simulink model "Example_MultiPID"  (R2017b)
settings: Solver=FixedStepAuto  StartTime=0.0  StopTime=inf  FixedStep=0.01  RelTol=1e-3  EnableMultiTasking=on
libraries: OBD2_SocketCan_Library x1
settings Model: SimulationMode=external  Creator=Murml  LastModifiedBy=Murml
settings SolverCC: PositivePriorityOrder=on
settings OptimizationCC: PassReuseOutputArgsThreshold=0  MaxStackSize=64
settings DebuggingCC: ParameterTunabilityLossMsg=error
settings HardwareCC: ProdBitPerPointer=32  ProdBitPerSizeT=32  ProdBitPerPtrDiffT=32  ProdLargestAtomicInteger=Long  ProdLargestAtomicFloat=Double  ProdWordSize=32  ProdHWDeviceType=ARM Compatible->ARM Cortex  UseEmbeddedCoderFeatures=off
settings SFSimCC: MATLABDynamicMemAlloc=off
settings RTWCC: SystemTargetFile=ert.tlc  HardwareBoard=Raspberry Pi  TemplateMakefile=ert_default_tmf  Toolchain=GNU GCC Raspberry Pi
settings CodeAppCC: ForceParamTrailComments=on  OperatorAnnotations=on
settings ERTTargetCC: ERTCustomFileBanners=off  SupportContinuousTime=on  SupportNonInlinedSFcns=on  RemoveResetFunc=off  SupportVariableSizeSignals=on  ModelStepFunctionPrototypeControlCompliant=off

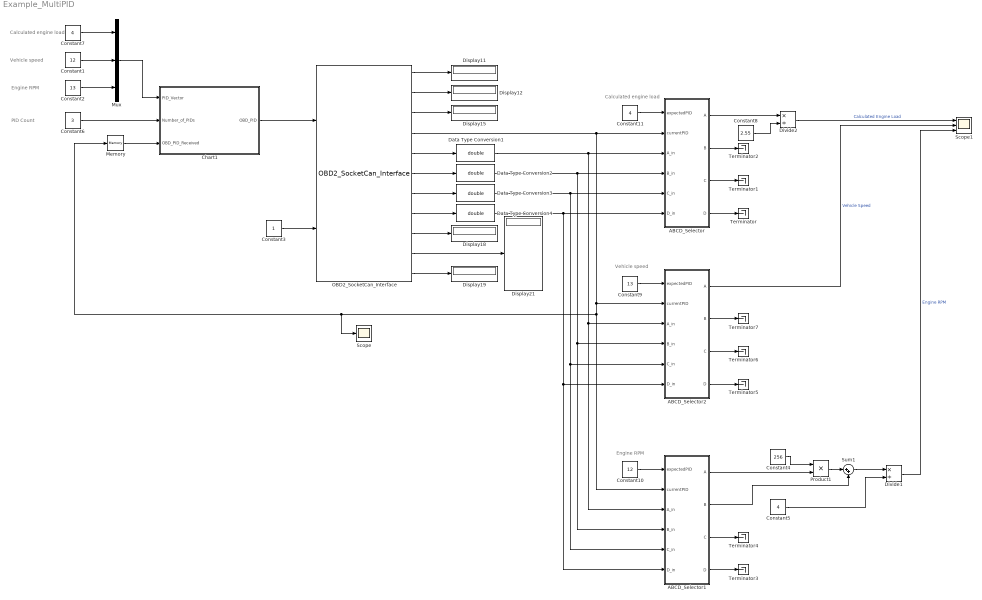
== system Example_MultiPID ==
  note: Calculated engine load
  note: Vehicle speed
  note: Engine RPM
  note: PID Count
  note: Calculated engine load
  note: Engine RPM
  note: Vehicle speed
  ABCD_Selector : MATLAB Function  TreatAsAtomicUnit=on
  ABCD_Selector1 : MATLAB Function  TreatAsAtomicUnit=on
  ABCD_Selector2 : MATLAB Function  TreatAsAtomicUnit=on
  Chart1 : Stateflow chart  TreatAsAtomicUnit=on
  Constant1 : Constant  Value=12  OutDataTypeStr=uint8  SampleTime=-1
  Constant10 : Constant  Value=12  OutDataTypeStr=uint8  SampleTime=-1
  Constant11 : Constant  Value=4  OutDataTypeStr=uint8  SampleTime=-1
  Constant2 : Constant  Value=13  OutDataTypeStr=uint8  SampleTime=-1
  Constant3 : Constant  OutDataTypeStr=uint8  SampleTime=-1
  Constant4 : Constant  Value=256  SampleTime=-1
  Constant5 : Constant  Value=4  SampleTime=-1
  Constant6 : Constant  Value=3  OutDataTypeStr=uint8  SampleTime=-1
  Constant7 : Constant  Value=4  OutDataTypeStr=uint8  SampleTime=-1
  Constant8 : Constant  Value=2.55  SampleTime=-1
  Constant9 : Constant  Value=13  OutDataTypeStr=uint8  SampleTime=-1
  Data Type Conversion{1..4} (4 alike) : DataTypeConversion  OutDataTypeStr=double
  Display{11..12,15,18..19,21} (6 alike) : Display
      Display11 settings: Format=hex (Stored Integer)
  Divide1 : Product  Inputs=*/
  Divide2 : Product  Inputs=*/
  Memory : Memory
  Mux : Mux  Inputs=3
  OBD2_SocketCan_Interface : OBD2_SocketCan_Library/OBD2_SocketCan_Interface  sampleTime=0.1
      settings: SourceProductName=OBD2 SocketCan Interface
  Product1 : Product
  Scope : Scope
  Scope1 : Scope  NumInputPorts=3
  Sum1 : Sum  Inputs=|++
  Terminator{,1..7} (8 alike) : Terminator
  wires:
  Constant3/1 -> OBD2_SocketCan_Interface/2
  OBD2_SocketCan_Interface/3 -> Display15/1
  OBD2_SocketCan_Interface/9 -> Display18/1
  Constant5/1 -> Divide1/2
  OBD2_SocketCan_Interface/1 -> Display11/1
  OBD2_SocketCan_Interface/2 -> Display12/1
  Sum1/1 -> Divide1/1
  Product1/1 -> Sum1/1
  Constant4/1 -> Product1/1
  OBD2_SocketCan_Interface/7 -> Data Type Conversion3/1
  OBD2_SocketCan_Interface/8 -> Data Type Conversion4/1
  OBD2_SocketCan_Interface/11 -> Display19/1
  OBD2_SocketCan_Interface/10 -> Display21/1
  Chart1/1(OBD_PID) -> OBD2_SocketCan_Interface/1
  Constant6/1 -> Chart1/2(Number_of_PIDs)
  Memory/1 -> Chart1/3(OBD_PID_Received)
  Mux/1 -> Chart1/1(PID_Vector)
  Constant2/1 -> Mux/3
  Constant1/1 -> Mux/2
  Constant7/1 -> Mux/1
  Constant8/1 -> Divide2/2
  Constant11/1 -> ABCD_Selector/1(expectedPID)
  OBD2_SocketCan_Interface/6 -> Data Type Conversion2/1
  OBD2_SocketCan_Interface/5 -> Data Type Conversion1/1
  ABCD_Selector/4(D) -> Terminator/1
  ABCD_Selector/3(C) -> Terminator1/1
  ABCD_Selector/2(B) -> Terminator2/1
  ABCD_Selector/1(A) -> Divide2/1
  Divide2/1 -> Scope1/1  "Calculated Engine Load"
  ABCD_Selector1/3(C) -> Terminator4/1
  ABCD_Selector1/4(D) -> Terminator3/1
  ABCD_Selector1/1(A) -> Product1/2
  ABCD_Selector1/2(B) -> Sum1/2
  Divide1/1 -> Scope1/3  "Engine RPM"
  ABCD_Selector2/3(C) -> Terminator6/1
  ABCD_Selector2/4(D) -> Terminator5/1
  ABCD_Selector2/2(B) -> Terminator7/1
  Constant10/1 -> ABCD_Selector1/1(expectedPID)
  Constant9/1 -> ABCD_Selector2/1(expectedPID)
  ABCD_Selector2/1(A) -> Scope1/2  "Vehicle Speed"
  OBD2_SocketCan_Interface/4 -> ABCD_Selector2/2(currentPID), ABCD_Selector1/2(currentPID), Scope/1, Memory/1, ABCD_Selector/2(currentPID)
  Data Type Conversion1/1 -> ABCD_Selector2/3(A_in), ABCD_Selector1/3(A_in), ABCD_Selector/3(A_in)
  Data Type Conversion2/1 -> ABCD_Selector2/4(B_in), ABCD_Selector1/4(B_in), ABCD_Selector/4(B_in)
  Data Type Conversion3/1 -> ABCD_Selector2/5(C_in), ABCD_Selector1/5(C_in), ABCD_Selector/5(C_in)
  Data Type Conversion4/1 -> ABCD_Selector/6(D_in), ABCD_Selector2/6(D_in), ABCD_Selector1/6(D_in)

== stateflow chart Example_MultiPID/Chart1 ==
  state INIT
    entry: currentPID = PID_Vector(1);
    OBD_PID = currentPID;
    pidCount = 1;
  state ResetCount
    entry: pidCount = 1;
    OBD_PID = PID_Vector(pidCount);
  state ChangePID
    entry:  pidCount = pidCount + 1;
    OBD_PID = PID_Vector(pidCount);
  (default) -> INIT
  INIT -> (junction 9) : [Number_of_PIDs > 1 && currentPID == OBD_PID_Received]
  ChangePID -> (junction 9)
  ResetCount -> (junction 9)
  (junction 9) -> ChangePID [order 1] : [pidCount < Number_of_PIDs]
  (junction 9) -> ResetCount [order 2] : [ pidCount >= Number_of_PIDs]
  data: PID_Vector input uint8; Number_of_PIDs input uint8; OBD_PID_Received input; OBD_PID output; pidCount local uint8; currentPID local uint8

== matlab function Example_MultiPID/ABCD_Selector ==
  data: expectedPID input; A output; currentPID input; B output; C output; D output; A_in input; B_in input; C_in input; D_in input
function [A,B,C,D]= fcn(expectedPID, currentPID, A_in , B_in, C_in, D_in)

% persistent variables
persistent A_OLD
persistent B_OLD
persistent C_OLD
persistent D_OLD

% variable init
if isempty(A_OLD)
	A_OLD = 0;
    B_OLD = 0;
    C_OLD = 0;
    D_OLD = 0;
end

% Use new data if available
if currentPID == expectedPID 
    A_OLD = A_in;
    B_OLD = B_in;
    C_OLD = C_in;
    D_OLD = D_in;   
end

% Output
A = A_OLD;
B = B_OLD;
C = C_OLD;
D = D_OLD;

== matlab function Example_MultiPID/ABCD_Selector1 ==
  data: expectedPID input; A output; currentPID input; B output; C output; D output; A_in input; B_in input; C_in input; D_in input
function [A,B,C,D]= fcn(expectedPID, currentPID, A_in , B_in, C_in, D_in)

% persistent variables
persistent A_OLD
persistent B_OLD
persistent C_OLD
persistent D_OLD

% variable init
if isempty(A_OLD)
	A_OLD = 0;
    B_OLD = 0;
    C_OLD = 0;
    D_OLD = 0;
end

% Use new data if available
if currentPID == expectedPID 
    A_OLD = A_in;
    B_OLD = B_in;
    C_OLD = C_in;
    D_OLD = D_in;   
end

% Output
A = A_OLD;
B = B_OLD;
C = C_OLD;
D = D_OLD;

== matlab function Example_MultiPID/ABCD_Selector2 ==
  data: expectedPID input; A output; currentPID input; B output; C output; D output; A_in input; B_in input; C_in input; D_in input
function [A,B,C,D]= fcn(expectedPID, currentPID, A_in , B_in, C_in, D_in)

% persistent variables
persistent A_OLD
persistent B_OLD
persistent C_OLD
persistent D_OLD

% variable init
if isempty(A_OLD)
	A_OLD = 0;
    B_OLD = 0;
    C_OLD = 0;
    D_OLD = 0;
end

% Use new data if available
if currentPID == expectedPID 
    A_OLD = A_in;
    B_OLD = B_in;
    C_OLD = C_in;
    D_OLD = D_in;   
end

% Output
A = A_OLD;
B = B_OLD;
C = C_OLD;
D = D_OLD;
